simulink model "Exemplo1"  (R2021a)
settings: Solver=VariableStepAuto  StartTime=0.0  StopTime=10.0  RelTol=1e-3
values from neighbouring files (symbols this model uses):
  A = [2 -3; 4 -5]    [script.m]
  B = [2 3; 4 -3]    [script.m]
  C = [1 5]    [script.m]
  D = [0 0]    [script.m]
settings Model: Creator=taffarel55  LastModifiedBy=taffarel55

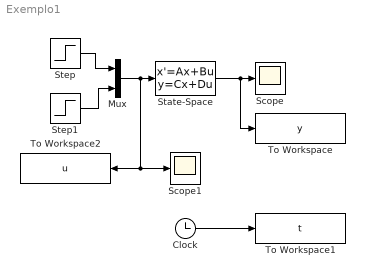
== system Exemplo1 ==
  Clock : Clock
  Mux : Mux  Inputs=2
  Scope : Scope
  Scope1 : Scope
  State-Space : StateSpace  A=A  B=B  C=C  D=D  InitialCondition=0
  Step : Step  Time=0  SampleTime=0
  Step1 : Step  Time=5  SampleTime=0
  To Workspace : ToWorkspace  VariableName=y  SaveFormat=Timeseries  SampleTime=-1
  To Workspace1 : ToWorkspace  VariableName=t  SaveFormat=Timeseries  SampleTime=-1
  To Workspace2 : ToWorkspace  VariableName=u  SaveFormat=Timeseries  SampleTime=-1
  wires:
  Mux/1 -> To Workspace2/1, Scope1/1, State-Space/1
  Step/1 -> Mux/1
  Step1/1 -> Mux/2
  State-Space/1 -> To Workspace/1, Scope/1
  Clock/1 -> To Workspace1/1
